simulink model "AM_System_Group5"  (R2024b)
settings: Solver=FixedStepAuto  StartTime=0.0  StopTime=100  FixedStep=1e-5  RelTol=1e-3
libraries: commchan3 x1, dspfdesign x1, dspstat3 x1, simulink x1
settings Model: Creator=lenovo  LastModifiedBy=lenovo

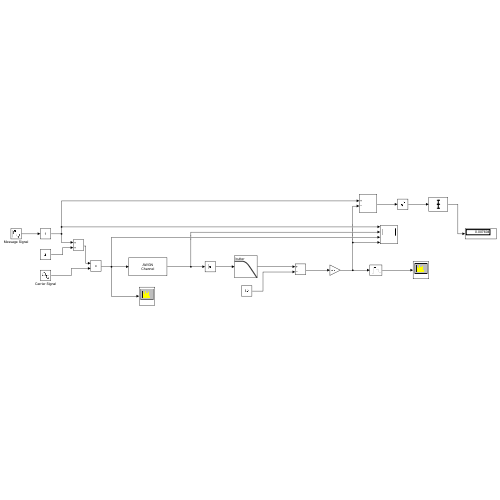
[thumbnail: Simulink's stored preview of the top-level diagram]
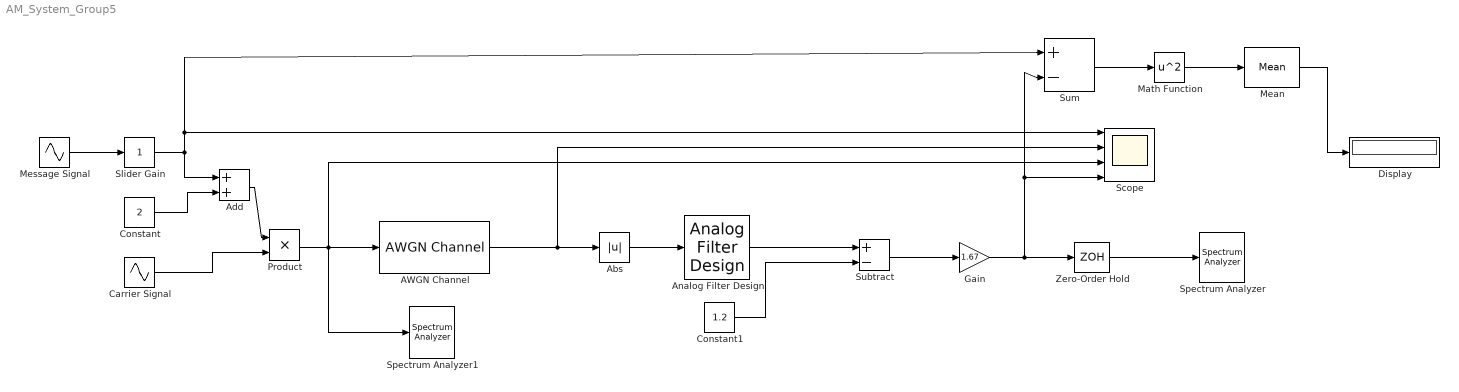
== system AM_System_Group5 ==
  AWGN Channel : commchan3/AWGN Channel  LegacyMode=off  NoiseMethod="Signal to noise ratio  (SNR)"  noiseMode="Signal to noise ratio  (SNR)"  EbNo=10  EsNo=10  SNR=20  BitsPerSymbol=1  SignalPower=1  SamplesPerSymbol=1  SymbolPeriod=1  VarianceSource=Parameter  Variance=1  RandomStream=Global stream  Seed=67  SimulateUsing=Code generation
  Abs : Abs  SaturateOnIntegerOverflow=off
  Add : Sum
  Analog Filter Design : dspfdesign/Analog Filter Design  method=Butterworth  filttype=Lowpass  N=2  Wlo=2*pi*50  Whi=80  Rp=2  Rs=40
  Carrier Signal : Sin  Frequency=2*pi*1000  SampleTime=0.0001
  Constant : Constant  Value=2
  Constant1 : Constant  Value=1.2
  Display : Display
  Gain : Gain  Gain=1.67
  Math Function : Math  Operator=square
  Mean : dspstat3/Mean  run=off  InputProcessing=Columns as channels (frame based)  reset_popup=None  directionMode=Each column  dimension=1  roiEnable=off  roiType=Rectangles  roiPortion=Entire ROI  roiOutput=Individual statistics for each ROI  roiFlag=off  roundingMode=Floor  overflowMode=off  outputDataTypeStr=Inherit: Same as accumulator  outputMin=[]  outputMax=[]  outputLastDataTypeStr=Inherit: Same as accumulator
  Message Signal : Sin  Frequency=2*pi*5  SampleTime=0.0001
  Product : Product
  Scope : Scope  NumInputPorts=4
  Slider Gain : simulink/Math Operations/Slider Gain  gain=1  low=0  high=2
  Spectrum Analyzer : SpectrumAnalyzer  WindowPosition=[447.000000,295.000000,800.000000,500.000000,]  ScopeFrameLocation=window  PlotAsTwoSidedSpectrum=off  WindowInvariantSamplesPerUpdate=on  FrequencySpan=Start and stop frequencies  Span=5000  CenterFrequency=2500  StartFrequency=0  StopFrequency=100  YLimits=[-37.21870480480443,50.470157739642474]  SelectedToolstripTab=spectrumAnalyzerToolstrip.estimationTab
  Spectrum Analyzer1 : SpectrumAnalyzer  WindowPosition=[293.000000,151.000000,800.000000,500.000000,]  ScopeFrameLocation=window  WindowInvariantSamplesPerUpdate=on  FrequencySpan=Start and stop frequencies  StartFrequency=900  StopFrequency=1100  YLimits=[-56.355662722897094,75.63349206592956]  SelectedToolstripTab=spectrumAnalyzerToolstrip.estimationTab
  Subtract : Sum  Inputs=+-
  Sum : Sum  Inputs=|+-|
  Zero-Order Hold : ZeroOrderHold  SampleTime=0.0001
  wires:
  Add/1 -> Product/1
  Carrier Signal/1 -> Product/2
  Product/1 -> Scope/3, Spectrum Analyzer1/1, AWGN Channel/1
  AWGN Channel/1 -> Scope/2, Abs/1
  Constant/1 -> Add/2
  Sum/1 -> Math Function/1
  Math Function/1 -> Mean/1
  Mean/1 -> Display/1
  Constant1/1 -> Subtract/2
  Abs/1 -> Analog Filter Design/1
  Analog Filter Design/1 -> Subtract/1
  Message Signal/1 -> Slider Gain/1
  Slider Gain/1 -> Add/1, Sum/1, Scope/1
  Subtract/1 -> Gain/1
  Gain/1 -> Zero-Order Hold/1, Sum/2, Scope/4
  Zero-Order Hold/1 -> Spectrum Analyzer/1
